simulink model "CommandMessage"  (R2024a)
settings: Solver=FixedStepAuto  StartTime=0.0  StopTime=0  FixedStep=0.01  RelTol=1e-3  EnableMultiTasking=on
undefined symbols (not defined in the file): actuatorCommand, allocationCommand, commandMode, ready, timestampUTC, useXNAllocation
libraries: MESSIN_Library x3
settings Model: Creator=damerius  LastModifiedBy=Scythe
settings SolverCC: ConcurrentTasks=on  AlgebraicLoopSolver=TrustRegion  PositivePriorityOrder=on
settings DataIOCC: SaveOutput=off  SignalLogging=off  DSMLogging=off  SaveTime=off  ReturnWorkspaceOutputs=off
settings OptimizationCC: DefaultParameterBehavior=Inlined  ReuseModelBlockBuffer=off  ZeroExternalMemoryAtStartup=off  ZeroInternalMemoryAtStartup=off  SimCompilerOptimization=on
settings DebuggingCC: UnconnectedInputMsg=warning  UnconnectedOutputMsg=warning  UnconnectedLineMsg=warning
settings HardwareCC: ProdBitPerLong=64  ProdHWDeviceType=Intel->x86-64 (Linux 64)
settings ModelReferenceCC: EnableRefExpFcnMdlSchedulingChecks=on
settings SFSimCC: SimParseCustomCode=off  SimGenImportedTypeDefs=on  SimTargetLang=C++
settings RTWCC: GenCodeOnly=on  PackageGeneratedCodeAndArtifacts=on  PackageName=PackNGo  RTWVerbose=off  BuildConfiguration=Faster Runs  TargetLang=C++  GPUComputeCapability=3.5  DLArmComputeVersion=19.05
settings CodeAppCC: ForceParamTrailComments=on  MaxIdLength=95  MATLABSourceComments=on  UseSimReservedNames=on
settings GRTTargetCC: TargetLangStandard=C++11 (ISO)  GenerateFullHeader=off  MatFileLogging=off  CodeInterfacePackaging=C++ class

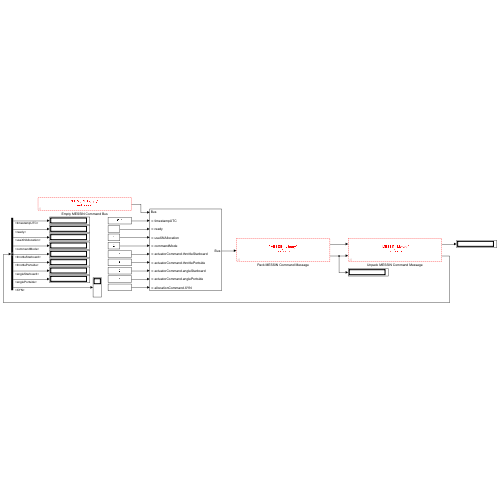
[thumbnail: Simulink's stored preview of the top-level diagram]
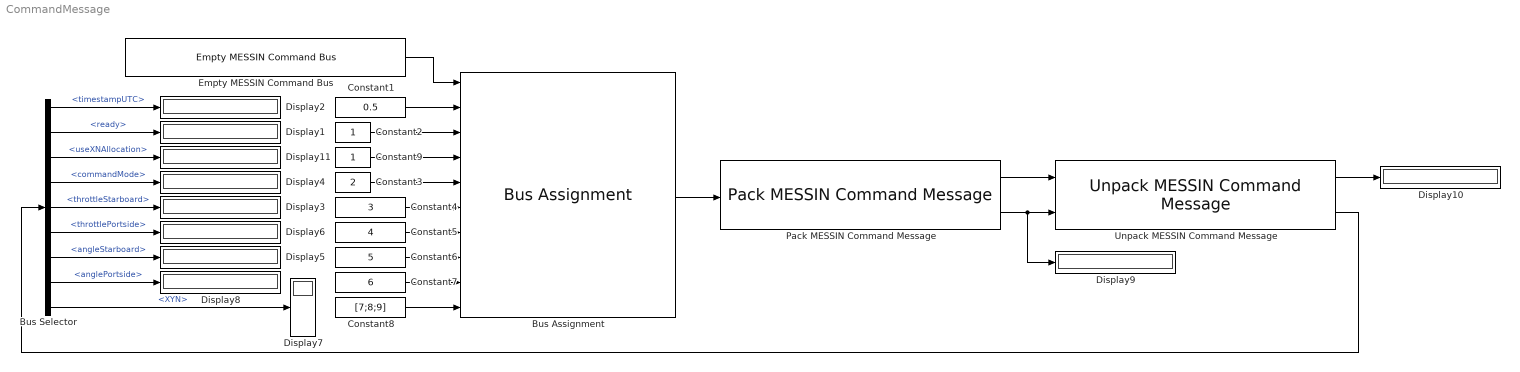
== system CommandMessage ==
  Bus Assignment : BusAssignment  AssignedSignals=timestampUTC,ready,useXNAllocation,commandMode,actuatorCommand.throttleStarboard,actuatorCommand.throttlePortside,actuatorCommand.angleStarboard,actuatorCommand.anglePortside,allocationCommand.XYN
  Bus Selector : BusSelector  OutputSignals=timestampUTC,ready,useXNAllocation,commandMode,actuatorCommand.throttleStarboard,actuatorCommand.throttlePortside,actuatorCommand.angleStarboard,actuatorCommand.anglePortside,allocationCommand.XYN
  Constant1 : Constant  Value=0.5  OutDataTypeStr=double
  Constant2 : Constant  OutDataTypeStr=boolean
  Constant3 : Constant  Value=2  OutDataTypeStr=uint8
  Constant4 : Constant  Value=3  OutDataTypeStr=double
  Constant5 : Constant  Value=4  OutDataTypeStr=double
  Constant6 : Constant  Value=5  OutDataTypeStr=double
  Constant7 : Constant  Value=6  OutDataTypeStr=double
  Constant8 : Constant  Value=[7;8;9]  OutDataTypeStr=double
  Constant9 : Constant  OutDataTypeStr=boolean
  Display{1..11} (11 alike) : Display
  Empty MESSIN Command Bus : MESSIN_Library/Command Message/Empty MESSIN Command Bus
      settings: SourceProductName=MESSIN - Interface Library
  Pack MESSIN Command Message : MESSIN_Library/Command Message/Pack MESSIN Command Message
      settings: SourceProductName=MESSIN - Interface Library
  Unpack MESSIN Command Message : MESSIN_Library/Command Message/Unpack MESSIN Command Message
      settings: SourceProductName=MESSIN - Interface Library
  wires:
  Constant9/1 -> Bus Assignment/4
  Bus Selector/3 -> Display11/1  "<useXNAllocation>"
  Bus Selector/7 -> Display5/1  "<angleStarboard>"
  Bus Selector/9 -> Display7/1  "<XYN>"
  Bus Selector/8 -> Display8/1  "<anglePortside>"
  Bus Selector/6 -> Display6/1  "<throttlePortside>"
  Bus Selector/5 -> Display3/1  "<throttleStarboard>"
  Bus Selector/4 -> Display4/1  "<commandMode>"
  Bus Selector/2 -> Display1/1  "<ready>"
  Bus Selector/1 -> Display2/1  "<timestampUTC>"
  Unpack MESSIN Command Message/2 -> Bus Selector/1
  Unpack MESSIN Command Message/1 -> Display10/1
  Pack MESSIN Command Message/2 -> Display9/1, Unpack MESSIN Command Message/2
  Pack MESSIN Command Message/1 -> Unpack MESSIN Command Message/1
  Bus Assignment/1 -> Pack MESSIN Command Message/1
  Constant8/1 -> Bus Assignment/10
  Constant7/1 -> Bus Assignment/9
  Constant6/1 -> Bus Assignment/8
  Constant5/1 -> Bus Assignment/7
  Constant4/1 -> Bus Assignment/6
  Constant3/1 -> Bus Assignment/5
  Constant2/1 -> Bus Assignment/3
  Constant1/1 -> Bus Assignment/2
  Empty MESSIN Command Bus/1 -> Bus Assignment/1
